simulink model "LSM_4p6U10_v01_06022022_NEW_ECC_2019a"  (R2019a)
settings: Solver=FixedStepAuto  StartTime=0.0  StopTime=Inf  FixedStep=Ts_lowspeed  RelTol=1e-3  EnableMultiTasking=on
PostLoadFcn:
  | , if any(exist('dsrtsu_mdlpostloadfcn', 'file') == [2, 3, 6]), try dsrtsu_mdlpostloadfcn('Execute', bdroot); catch fprintf('Error in PostLoadFcn (dsrtsu_mdlpostloadfcn) for model "%s":\n %s\n', bdroot, lasterr); end, end,
values from neighbouring files (symbols this model uses):
  Ts_lowspeed = 0.05    [Parameters_4p6U10.m]
undefined symbols (not defined in the file or in its folder): Down, GPTRIP1SEL, GPTRIP2SEL, TZ1, TZ2, Up
libraries: simulink x91, simulink_extras x25, c2802xlib x12, c2837xDlib x8, c280xlib x8
(part 2 of 2)

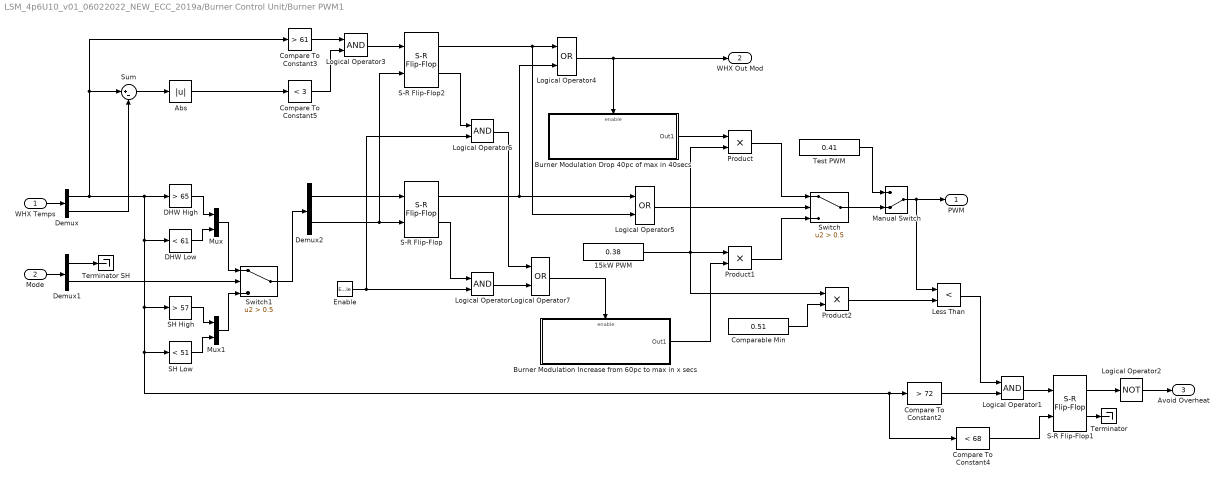
== system LSM_4p6U10_v01_06022022_NEW_ECC_2019a/Burner Control Unit/Burner PWM1 ==
  WHX Temps : Inport
  Mode : Inport  Port=2
  Enable : EnablePort  StatesWhenEnabling=reset  ShowOutputPort=on
  15kW PWM : Constant  Value=0.38  OutDataTypeStr=double
  Abs : Abs
  Burner Modulation Drop 40pc of max in 40secs : Subsystem
  Burner Modulation Increase from 60pc to max in x secs : Subsystem
  Comparable Min : Constant  Value=0.51  OutDataTypeStr=double
  Compare To Constant2 : simulink/Logic and Bit Operations/Compare To Constant  relop=>  const=72  OutDataTypeStr=boolean
  Compare To Constant3 : simulink/Logic and Bit Operations/Compare To Constant  relop=>  const=61  OutDataTypeStr=boolean
  Compare To Constant4 : simulink/Logic and Bit Operations/Compare To Constant  relop=<  const=68  OutDataTypeStr=boolean
  Compare To Constant5 : simulink/Logic and Bit Operations/Compare To Constant  relop=<  const=3  OutDataTypeStr=boolean
  DHW High : simulink/Logic and Bit Operations/Compare To Constant  relop=>  const=65  OutDataTypeStr=boolean
  DHW Low : simulink/Logic and Bit Operations/Compare To Constant  relop=<  const=61  OutDataTypeStr=boolean
  Demux : Demux  Outputs=2
  Demux1 : Demux  Outputs=2
  Demux2 : Demux  Outputs=2
  Less Than : RelationalOperator  Operator=<  OutDataTypeStr=boolean  RndMeth=Simplest
  Logical Operator{,1,3,6} (4 alike) : Logic  AllPortsSameDT=off  OutDataTypeStr=boolean
  Logical Operator2 : Logic  Operator=NOT  AllPortsSameDT=off  OutDataTypeStr=boolean
  Logical Operator4 : Logic  Operator=OR  AllPortsSameDT=off  OutDataTypeStr=boolean
  Logical Operator5 : Logic  Operator=OR  AllPortsSameDT=off  OutDataTypeStr=boolean
  Logical Operator7 : Logic  Operator=OR  AllPortsSameDT=off  OutDataTypeStr=boolean
  Manual Switch : ManualSwitch  CurrentSetting=0
  Mux : Mux  Inputs=2
  Mux1 : Mux  Inputs=2
  Product : Product
  Product1 : Product
  Product2 : Product
  S-R Flip-Flop : simulink_extras/Flip Flops/S-R Flip-Flop  initial_condition=0
  S-R Flip-Flop1 : simulink_extras/Flip Flops/S-R Flip-Flop  initial_condition=0
  S-R Flip-Flop2 : simulink_extras/Flip Flops/S-R Flip-Flop  initial_condition=0
  SH High : simulink/Logic and Bit Operations/Compare To Constant  relop=>  const=57  OutDataTypeStr=boolean
  SH Low : simulink/Logic and Bit Operations/Compare To Constant  relop=<  const=51  OutDataTypeStr=boolean
  Sum : Sum  Inputs=|+-
  Switch : Switch  Criteria=u2 > Threshold  Threshold=0.5
  Switch1 : Switch  Criteria=u2 > Threshold  Threshold=0.5
  Terminator : Terminator
  Terminator SH : Terminator
  Test PWM : Constant  Value=0.41  OutDataTypeStr=double
  PWM : Outport  VectorParamsAs1DForOutWhenUnconnected=on
  WHX Out Mod : Outport  Port=2  VectorParamsAs1DForOutWhenUnconnected=on
  Avoid Overheat : Outport  Port=3  VectorParamsAs1DForOutWhenUnconnected=on
  wires:
  Product2/1 -> Less Than/2
  Comparable Min/1 -> Product2/2
  Compare To Constant4/1 -> S-R Flip-Flop1/2
  Logical Operator2/1 -> Avoid Overheat/1
  S-R Flip-Flop1/1 -> Logical Operator2/1
  S-R Flip-Flop1/2 -> Terminator/1
  Logical Operator1/1 -> S-R Flip-Flop1/1
  Less Than/1 -> Logical Operator1/1
  Compare To Constant2/1 -> Logical Operator1/2
  Test PWM/1 -> Manual Switch/1
  Switch/1 -> Manual Switch/2
  Logical Operator/1 -> Logical Operator7/2
  Enable/1 -> Logical Operator6/2, Logical Operator/2
  Product1/1 -> Switch/3
  Burner Modulation Increase from 60pc to max in x secs/1(Out1) -> Product1/2
  Product/1 -> Switch/1
  Burner Modulation Drop 40pc of max in 40secs/1(Out1) -> Product/1
  Demux2/2 -> S-R Flip-Flop2/2, S-R Flip-Flop/2
  Manual Switch/1 -> PWM/1, Less Than/1
  S-R Flip-Flop/2 -> Logical Operator/1
  S-R Flip-Flop/1 -> Logical Operator5/1, Logical Operator4/2
  Demux2/1 -> S-R Flip-Flop/1
  Demux/1 -> DHW High/1, DHW Low/1, Compare To Constant2/1, Compare To Constant4/1, SH Low/1, SH High/1, Compare To Constant3/1, Sum/1
  15kW PWM/1 -> Product2/1, Product/2, Product1/1
  WHX Temps/1 -> Demux/1
  Demux/2 -> Sum/2
  Sum/1 -> Abs/1
  Abs/1 -> Compare To Constant5/1
  Compare To Constant3/1 -> Logical Operator3/1
  Compare To Constant5/1 -> Logical Operator3/2
  Logical Operator3/1 -> S-R Flip-Flop2/1
  S-R Flip-Flop2/1 -> Logical Operator5/2, Logical Operator4/1
  Logical Operator4/1 -> Burner Modulation Drop 40pc of max in 40secs/Enable, WHX Out Mod/1
  S-R Flip-Flop2/2 -> Logical Operator6/1
  Logical Operator5/1 -> Switch/2
  Logical Operator7/1 -> Burner Modulation Increase from 60pc to max in x secs/Enable
  Logical Operator6/1 -> Logical Operator7/1
  Mode/1 -> Demux1/1
  Demux1/1 -> Terminator SH/1
  Demux1/2 -> Switch1/2
  DHW High/1 -> Mux/1
  DHW Low/1 -> Mux/2
  SH High/1 -> Mux1/1
  SH Low/1 -> Mux1/2
  Mux1/1 -> Switch1/3
  Mux/1 -> Switch1/1
  Switch1/1 -> Demux2/1

== system LSM_4p6U10_v01_06022022_NEW_ECC_2019a/Burner Control Unit/Emergency Burner Shut Off ==
  Max HHT Temp : Inport
  Boolean 0 : Constant  Value=0  OutDataTypeStr=boolean
  Boolean 1 : Constant  OutDataTypeStr=boolean
  Boolean 14 : Constant  OutDataTypeStr=boolean
  Boolean 15 : Constant  Value=0  OutDataTypeStr=boolean
  Data Type Conversion : DataTypeConversion  OutDataTypeStr=double
  Emergency Shut Off T3 : Switch  Criteria=u2 > Threshold  Threshold=615
  Logical Operator : Logic  Operator=NOT  AllPortsSameDT=off  OutDataTypeStr=boolean
  S-R Flip-Flop : simulink_extras/Flip Flops/S-R Flip-Flop  initial_condition=0
  T3 Temp TH Reset : Switch  Criteria=u2 > Threshold  Threshold=450
  Terminator : Terminator
  Shut Off Command : Outport  VectorParamsAs1DForOutWhenUnconnected=on
  Emergency Shut OFF BL : Outport  Port=2  VectorParamsAs1DForOutWhenUnconnected=on
  wires:
  Boolean 1/1 -> Emergency Shut Off T3/1
  Boolean 0/1 -> Emergency Shut Off T3/3
  Emergency Shut Off T3/1 -> S-R Flip-Flop/1
  S-R Flip-Flop/1 -> Emergency Shut OFF BL/1, Logical Operator/1
  S-R Flip-Flop/2 -> Terminator/1
  T3 Temp TH Reset/1 -> S-R Flip-Flop/2
  Max HHT Temp/1 -> T3 Temp TH Reset/2, Emergency Shut Off T3/2
  Boolean 15/1 -> T3 Temp TH Reset/1
  Boolean 14/1 -> T3 Temp TH Reset/3
  Logical Operator/1 -> Data Type Conversion/1
  Data Type Conversion/1 -> Shut Off Command/1

== system LSM_4p6U10_v01_06022022_NEW_ECC_2019a/Burner Control Unit/Protected Modulation Drop 25pc of max in 50s ==
  Enable : EnablePort  StatesWhenEnabling=reset
  Constant : Constant
  Gain : Gain  Gain=-0.0025
  Integrator : Integrator  LimitOutput=on  UpperSaturationLimit=300  LowerSaturationLimit=0
  Limit Saturation : Saturate  UpperLimit=1  LowerLimit=0.75
  Sum : Sum  Inputs=|++
  Unit : Constant
  Out1 : Outport  VectorParamsAs1DForOutWhenUnconnected=on
  wires:
  Constant/1 -> Integrator/1
  Integrator/1 -> Gain/1
  Gain/1 -> Sum/1
  Unit/1 -> Sum/2
  Sum/1 -> Limit Saturation/1
  Limit Saturation/1 -> Out1/1

== system LSM_4p6U10_v01_06022022_NEW_ECC_2019a/Burner Control Unit/Reduction of Max PWM ==
  Max HHX Temp : Inport
  Boolean 0 : Constant  Value=0  OutDataTypeStr=boolean
  Boolean 1 : Constant  OutDataTypeStr=boolean
  Boolean 14 : Constant  OutDataTypeStr=boolean
  Boolean 15 : Constant  Value=0  OutDataTypeStr=boolean
  Emergency Shut Off T3 : Switch  Criteria=u2 > Threshold  Threshold=600
  S-R Flip-Flop : simulink_extras/Flip Flops/S-R Flip-Flop  initial_condition=0
  T3 Temp TH Reset : Switch  Criteria=u2 > Threshold  Threshold=580
  Terminator : Terminator
  Boolean 1 For Protection : Outport  VectorParamsAs1DForOutWhenUnconnected=on
  wires:
  Boolean 1/1 -> Emergency Shut Off T3/1
  Boolean 0/1 -> Emergency Shut Off T3/3
  Emergency Shut Off T3/1 -> S-R Flip-Flop/1
  S-R Flip-Flop/2 -> Terminator/1
  T3 Temp TH Reset/1 -> S-R Flip-Flop/2
  Max HHX Temp/1 -> T3 Temp TH Reset/2, Emergency Shut Off T3/2
  Boolean 15/1 -> T3 Temp TH Reset/1
  Boolean 14/1 -> T3 Temp TH Reset/3
  S-R Flip-Flop/1 -> Boolean 1 For Protection/1

== system LSM_4p6U10_v01_06022022_NEW_ECC_2019a/Flame Sense Relative to Motion/FLAME LOSS DECISION ==
  Enable : EnablePort  StatesWhenEnabling=reset
  0 to 91 : Integrator  LimitOutput=on  UpperSaturationLimit=91  LowerSaturationLimit=0
  Compare To Constant : simulink/Logic and Bit Operations/Compare To Constant  relop=>  const=90  OutDataTypeStr=boolean
  Constant : Constant
  Out1 : Outport
  wires:
  0 to 91/1 -> Compare To Constant/1
  Constant/1 -> 0 to 91/1
  Compare To Constant/1 -> Out1/1

== system LSM_4p6U10_v01_06022022_NEW_ECC_2019a/Pump Commands FIELD INSTALLATION/Conversion for micro ==
  WHXPC : Inport
  CHXPC : Inport  Port=2
  Ceil2 : Rounding  Operator=ceil
  Ceil4 : Rounding  Operator=ceil
  "Convert Volts to 0-1 Command " : Gain  Gain=1/10
  Convert Volts to 0-1 Command : Gain  Gain=1/10
  Convert to uint1 : DataTypeConversion  OutDataTypeStr=uint16
  Convert to uint16 : DataTypeConversion  OutDataTypeStr=uint16
  Gain2 : Gain  Gain=1023
  Gain3 : Gain  Gain=1023
  CHX Pump : Outport
  WHX Pump : Outport  Port=2
  wires:
  Ceil4/1 -> Convert to uint1/1
  Ceil2/1 -> Convert to uint16/1
  Convert to uint16/1 -> CHX Pump/1  "CHX Pump"
  Gain3/1 -> Ceil2/1
  Convert to uint1/1 -> WHX Pump/1  "WHX Pump"
  "Convert Volts to 0-1 Command "/1 -> Gain2/1
  Convert Volts to 0-1 Command/1 -> Gain3/1
  CHXPC/1 -> "Convert Volts to 0-1 Command "/1
  Gain2/1 -> Ceil4/1
  WHXPC/1 -> Convert Volts to 0-1 Command/1

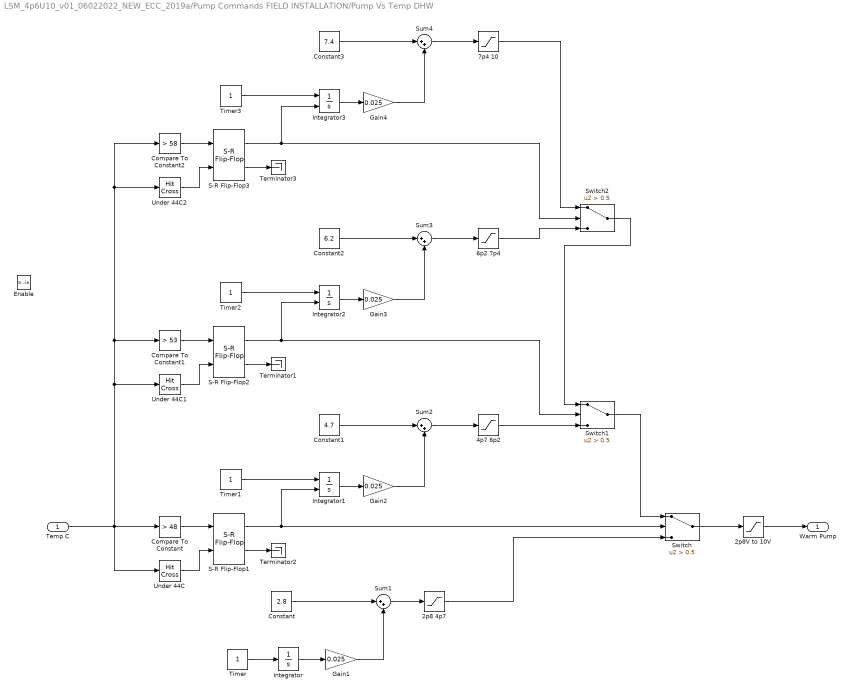
== system LSM_4p6U10_v01_06022022_NEW_ECC_2019a/Pump Commands FIELD INSTALLATION/Pump Vs Temp DHW ==
  Temp C : Inport
  Enable : EnablePort  StatesWhenEnabling=reset
  2p8 4p7 : Saturate  UpperLimit=4.7  LowerLimit=2.8
  2p8V to 10V : Saturate  UpperLimit=10  LowerLimit=2.8
  4p7 6p2 : Saturate  UpperLimit=6.2  LowerLimit=4.7
  6p2 7p4 : Saturate  UpperLimit=7.4  LowerLimit=6.2
  7p4 10 : Saturate  UpperLimit=10  LowerLimit=7.4
  Compare To Constant : simulink/Logic and Bit Operations/Compare To Constant  relop=>  const=48  OutDataTypeStr=boolean
  Compare To Constant1 : simulink/Logic and Bit Operations/Compare To Constant  relop=>  const=53  OutDataTypeStr=boolean
  Compare To Constant2 : simulink/Logic and Bit Operations/Compare To Constant  relop=>  const=58  OutDataTypeStr=boolean
  Constant : Constant  Value=2.8
  Constant1 : Constant  Value=4.7
  Constant2 : Constant  Value=6.2
  Constant3 : Constant  Value=7.4
  Gain{1..4} (4 alike) : Gain  Gain=0.025
  Integrator : Integrator  LimitOutput=on  UpperSaturationLimit=300  LowerSaturationLimit=0
  Integrator1 : Integrator  ExternalReset=rising  LimitOutput=on  UpperSaturationLimit=300  LowerSaturationLimit=0
  Integrator2 : Integrator  ExternalReset=rising  LimitOutput=on  UpperSaturationLimit=300  LowerSaturationLimit=0
  Integrator3 : Integrator  ExternalReset=rising  LimitOutput=on  UpperSaturationLimit=300  LowerSaturationLimit=0
  S-R Flip-Flop1 : simulink_extras/Flip Flops/S-R Flip-Flop  initial_condition=0
  S-R Flip-Flop2 : simulink_extras/Flip Flops/S-R Flip-Flop  initial_condition=0
  S-R Flip-Flop3 : simulink_extras/Flip Flops/S-R Flip-Flop  initial_condition=0
  Sum{1..4} (4 alike) : Sum  Inputs=|++
  Switch : Switch  Criteria=u2 > Threshold  Threshold=0.5
  Switch1 : Switch  Criteria=u2 > Threshold  Threshold=0.5
  Switch2 : Switch  Criteria=u2 > Threshold  Threshold=0.5
  Terminator1 : Terminator
  Terminator2 : Terminator
  Terminator3 : Terminator
  Timer{,1..3} (4 alike) : Constant
  Under 44C : HitCross  HitCrossingOffset=40  HitCrossingDirection=falling
  Under 44C1 : HitCross  HitCrossingOffset=40  HitCrossingDirection=falling
  Under 44C2 : HitCross  HitCrossingOffset=40  HitCrossingDirection=falling
  Warm Pump : Outport  VectorParamsAs1DForOutWhenUnconnected=on
  wires:
  2p8V to 10V/1 -> Warm Pump/1
  S-R Flip-Flop1/2 -> Terminator2/1
  Under 44C/1 -> S-R Flip-Flop1/2
  Compare To Constant/1 -> S-R Flip-Flop1/1
  S-R Flip-Flop1/1 -> Switch/2, Integrator1/2
  Constant/1 -> Sum1/1
  Gain1/1 -> Sum1/2
  Sum1/1 -> 2p8 4p7/1
  Integrator/1 -> Gain1/1
  Timer/1 -> Integrator/1
  2p8 4p7/1 -> Switch/3
  Gain2/1 -> Sum2/2
  Integrator1/1 -> Gain2/1
  Constant1/1 -> Sum2/1
  Timer1/1 -> Integrator1/1
  4p7 6p2/1 -> Switch1/3
  Sum2/1 -> 4p7 6p2/1
  Switch1/1 -> Switch/1
  Switch/1 -> 2p8V to 10V/1
  6p2 7p4/1 -> Switch2/3
  Sum3/1 -> 6p2 7p4/1
  Timer2/1 -> Integrator2/1
  Integrator2/1 -> Gain3/1
  S-R Flip-Flop2/1 -> Switch1/2, Integrator2/2
  S-R Flip-Flop2/2 -> Terminator1/1
  Compare To Constant1/1 -> S-R Flip-Flop2/1
  Constant2/1 -> Sum3/1
  Under 44C1/1 -> S-R Flip-Flop2/2
  Gain3/1 -> Sum3/2
  S-R Flip-Flop3/2 -> Terminator3/1
  Under 44C2/1 -> S-R Flip-Flop3/2
  S-R Flip-Flop3/1 -> Switch2/2, Integrator3/2
  Compare To Constant2/1 -> S-R Flip-Flop3/1
  Constant3/1 -> Sum4/1
  Sum4/1 -> 7p4 10/1
  Integrator3/1 -> Gain4/1
  7p4 10/1 -> Switch2/1
  Temp C/1 -> Compare To Constant2/1, Under 44C2/1, Compare To Constant1/1, Under 44C1/1, Under 44C/1, Compare To Constant/1
  Gain4/1 -> Sum4/2
  Timer3/1 -> Integrator3/1
  Switch2/1 -> Switch1/1

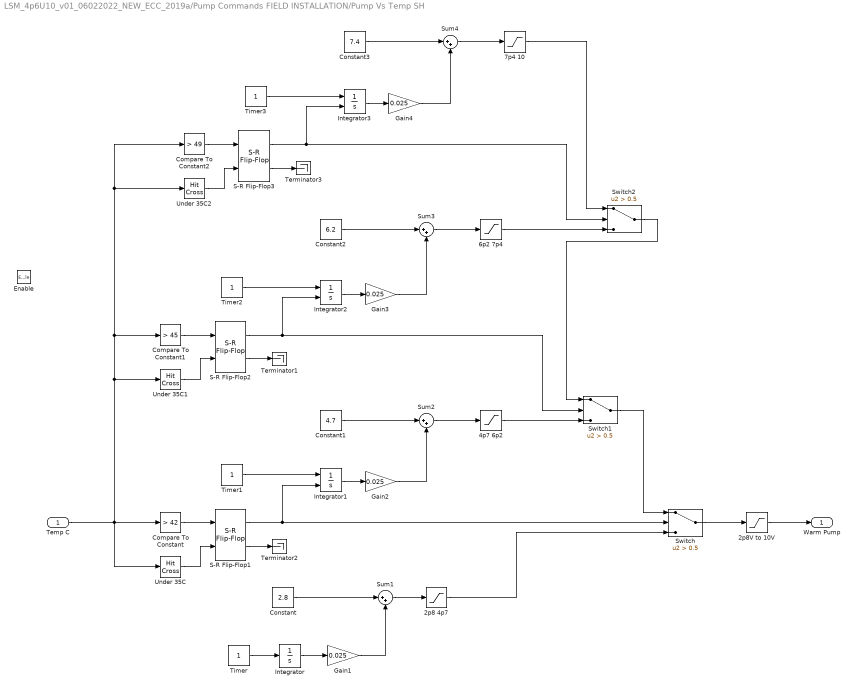
== system LSM_4p6U10_v01_06022022_NEW_ECC_2019a/Pump Commands FIELD INSTALLATION/Pump Vs Temp SH ==
  Temp C : Inport
  Enable : EnablePort  StatesWhenEnabling=reset
  2p8 4p7 : Saturate  UpperLimit=4.7  LowerLimit=2.8
  2p8V to 10V : Saturate  UpperLimit=10  LowerLimit=2.8
  4p7 6p2 : Saturate  UpperLimit=6.2  LowerLimit=4.7
  6p2 7p4 : Saturate  UpperLimit=7.4  LowerLimit=6.2
  7p4 10 : Saturate  UpperLimit=10  LowerLimit=7.4
  Compare To Constant : simulink/Logic and Bit Operations/Compare To Constant  relop=>  const=42  OutDataTypeStr=boolean
  Compare To Constant1 : simulink/Logic and Bit Operations/Compare To Constant  relop=>  const=45  OutDataTypeStr=boolean
  Compare To Constant2 : simulink/Logic and Bit Operations/Compare To Constant  relop=>  const=49  OutDataTypeStr=boolean
  Constant : Constant  Value=2.8
  Constant1 : Constant  Value=4.7
  Constant2 : Constant  Value=6.2
  Constant3 : Constant  Value=7.4
  Gain{1..4} (4 alike) : Gain  Gain=0.025
  Integrator : Integrator  LimitOutput=on  UpperSaturationLimit=300  LowerSaturationLimit=0
  Integrator1 : Integrator  ExternalReset=rising  LimitOutput=on  UpperSaturationLimit=300  LowerSaturationLimit=0
  Integrator2 : Integrator  ExternalReset=rising  LimitOutput=on  UpperSaturationLimit=300  LowerSaturationLimit=0
  Integrator3 : Integrator  ExternalReset=rising  LimitOutput=on  UpperSaturationLimit=300  LowerSaturationLimit=0
  S-R Flip-Flop1 : simulink_extras/Flip Flops/S-R Flip-Flop  initial_condition=0
  S-R Flip-Flop2 : simulink_extras/Flip Flops/S-R Flip-Flop  initial_condition=0
  S-R Flip-Flop3 : simulink_extras/Flip Flops/S-R Flip-Flop  initial_condition=0
  Sum{1..4} (4 alike) : Sum  Inputs=|++
  Switch : Switch  Criteria=u2 > Threshold  Threshold=0.5
  Switch1 : Switch  Criteria=u2 > Threshold  Threshold=0.5
  Switch2 : Switch  Criteria=u2 > Threshold  Threshold=0.5
  Terminator1 : Terminator
  Terminator2 : Terminator
  Terminator3 : Terminator
  Timer{,1..3} (4 alike) : Constant
  Under 35C : HitCross  HitCrossingOffset=35  HitCrossingDirection=falling
  Under 35C1 : HitCross  HitCrossingOffset=35  HitCrossingDirection=falling
  Under 35C2 : HitCross  HitCrossingOffset=35  HitCrossingDirection=falling
  Warm Pump : Outport  VectorParamsAs1DForOutWhenUnconnected=on
  wires:
  2p8V to 10V/1 -> Warm Pump/1
  S-R Flip-Flop1/2 -> Terminator2/1
  Under 35C/1 -> S-R Flip-Flop1/2
  Compare To Constant/1 -> S-R Flip-Flop1/1
  S-R Flip-Flop1/1 -> Switch/2, Integrator1/2
  Constant/1 -> Sum1/1
  Gain1/1 -> Sum1/2
  Sum1/1 -> 2p8 4p7/1
  Integrator/1 -> Gain1/1
  Timer/1 -> Integrator/1
  2p8 4p7/1 -> Switch/3
  Gain2/1 -> Sum2/2
  Integrator1/1 -> Gain2/1
  Constant1/1 -> Sum2/1
  Timer1/1 -> Integrator1/1
  4p7 6p2/1 -> Switch1/3
  Sum2/1 -> 4p7 6p2/1
  Switch1/1 -> Switch/1
  Switch/1 -> 2p8V to 10V/1
  6p2 7p4/1 -> Switch2/3
  Sum3/1 -> 6p2 7p4/1
  Timer2/1 -> Integrator2/1
  Integrator2/1 -> Gain3/1
  S-R Flip-Flop2/1 -> Switch1/2, Integrator2/2
  S-R Flip-Flop2/2 -> Terminator1/1
  Compare To Constant1/1 -> S-R Flip-Flop2/1
  Constant2/1 -> Sum3/1
  Under 35C1/1 -> S-R Flip-Flop2/2
  Gain3/1 -> Sum3/2
  Constant3/1 -> Sum4/1
  Gain4/1 -> Sum4/2
  7p4 10/1 -> Switch2/1
  Under 35C2/1 -> S-R Flip-Flop3/2
  Integrator3/1 -> Gain4/1
  S-R Flip-Flop3/1 -> Switch2/2, Integrator3/2
  Temp C/1 -> Compare To Constant2/1, Under 35C2/1, Compare To Constant1/1, Under 35C1/1, Under 35C/1, Compare To Constant/1
  Compare To Constant2/1 -> S-R Flip-Flop3/1
  S-R Flip-Flop3/2 -> Terminator3/1
  Sum4/1 -> 7p4 10/1
  Timer3/1 -> Integrator3/1
  Switch2/1 -> Switch1/1

== system LSM_4p6U10_v01_06022022_NEW_ECC_2019a/Pump Commands FIELD INSTALLATION/Timer // Integrator 0-101s1 ==
  WPC : Inport
  Enable : EnablePort  StatesWhenEnabling=reset  ShowOutputPort=on
  Gain : Gain  Gain=-0.1
  Integrator : Integrator  ExternalReset=rising  LimitOutput=on  UpperSaturationLimit=300  LowerSaturationLimit=0
  Saturation : Saturate  UpperLimit=10  LowerLimit=2.8
  Sum : Sum  Inputs=|++
  Timer : Constant
  Out1 : Outport  VectorParamsAs1DForOutWhenUnconnected=on
  wires:
  Timer/1 -> Integrator/1
  Integrator/1 -> Gain/1
  Enable/1 -> Integrator/2
  Sum/1 -> Saturation/1
  WPC/1 -> Sum/1
  Gain/1 -> Sum/2
  Saturation/1 -> Out1/1

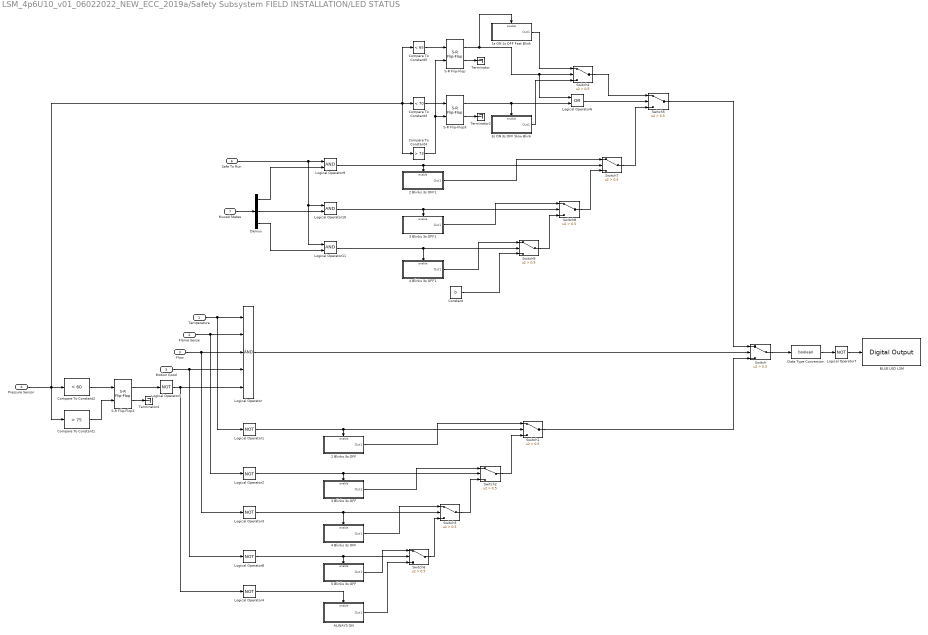
== system LSM_4p6U10_v01_06022022_NEW_ECC_2019a/Safety Subsystem FIELD INSTALLATION/LED STATUS ==
  Temperature : Inport
  Flame Sense : Inport  Port=2
  Flow : Inport  Port=3
  Pressure Sensor : Inport  Port=4
  Motion Good : Inport  Port=5
  Safe To Run : Inport  Port=6
  Muxed States : Inport  Port=7
  1s ON 1s OFF Fast Blink : Subsystem
  2 Blinks 3s OFF : Subsystem
  2 Blinks 3s OFF1 : Subsystem
  3 Blinks 3s OFF : Subsystem
  3 Blinks 3s OFF1 : Subsystem
  3s ON 3s OFF Slow Blink : Subsystem
  4 Blinks 3s OFF : Subsystem
  4 Blinks 3s OFF1 : Subsystem
  5 Blinks 3s OFF : Subsystem
  ALWAYS ON : Subsystem
  BLUE LED LSM : c2837xDlib/Digital Output  GPIO_Number=GPIO24~GPIO31  GPIO_Bit0=off  GPIO_BIT0_Toggle=off  GPIO_Bit1=off  GPIO_BIT1_Toggle=off  GPIO_Bit2=off  GPIO_BIT2_Toggle=off  GPIO_Bit3=off  GPIO_BIT3_Toggle=off  GPIO_Bit4=off  GPIO_BIT4_Toggle=off  GPIO_Bit5=off  GPIO_BIT5_Toggle=off  GPIO_Bit6=off  GPIO_BIT6_Toggle=off  GPIO_Bit7=on  GPIO_BIT7_Toggle=off
      settings: SourceProductBaseCode=TIC2000
  Compare To Constant1 : simulink/Logic and Bit Operations/Compare To Constant  relop=>  const=75  OutDataTypeStr=boolean
  Compare To Constant2 : simulink/Logic and Bit Operations/Compare To Constant  relop=<  const=60  OutDataTypeStr=boolean
  Compare To Constant3 : simulink/Logic and Bit Operations/Compare To Constant  relop=<  const=70  OutDataTypeStr=boolean
  Compare To Constant4 : simulink/Logic and Bit Operations/Compare To Constant  relop=>  const=73  OutDataTypeStr=boolean
  Compare To Constant5 : simulink/Logic and Bit Operations/Compare To Constant  relop=<  const=65  OutDataTypeStr=boolean
  Constant : Constant  Value=0  OutDataTypeStr=boolean
  Data Type Conversion : DataTypeConversion  OutDataTypeStr=boolean
  Demux : Demux  Outputs=3
  Logical Operator : Logic  Inputs=5  AllPortsSameDT=off  OutDataTypeStr=boolean
  Logical Operator{1..5,7..8} (7 alike) : Logic  Operator=NOT  AllPortsSameDT=off  OutDataTypeStr=boolean
  Logical Operator10 : Logic  AllPortsSameDT=off  OutDataTypeStr=boolean
  Logical Operator11 : Logic  AllPortsSameDT=off  OutDataTypeStr=boolean
  Logical Operator6 : Logic  Operator=OR  AllPortsSameDT=off  OutDataTypeStr=boolean
  Logical Operator9 : Logic  AllPortsSameDT=off  OutDataTypeStr=boolean
  S-R Flip-Flop : simulink_extras/Flip Flops/S-R Flip-Flop  initial_condition=0
  S-R Flip-Flop1 : simulink_extras/Flip Flops/S-R Flip-Flop  initial_condition=0
  S-R Flip-Flop3 : simulink_extras/Flip Flops/S-R Flip-Flop  initial_condition=0
  Switch{,1..9} (10 alike) : Switch  Criteria=u2 > Threshold  Threshold=0.5
  Terminator : Terminator
  Terminator2 : Terminator
  Terminator4 : Terminator
  wires:
  Temperature/1 -> Logical Operator1/1, Logical Operator/1
  Flame Sense/1 -> Logical Operator2/1, Logical Operator/2
  Flow/1 -> Logical Operator3/1, Logical Operator/3
  Logical Operator5/1 -> Logical Operator/5, Logical Operator4/1
  Logical Operator/1 -> Switch/2
  Logical Operator1/1 -> Switch1/2, 2 Blinks 3s OFF/Enable
  Logical Operator2/1 -> Switch2/2, 3 Blinks 3s OFF/Enable
  Logical Operator3/1 -> Switch3/2, 4 Blinks 3s OFF/Enable
  Logical Operator4/1 -> ALWAYS ON/Enable
  Compare To Constant1/1 -> S-R Flip-Flop1/2
  Compare To Constant2/1 -> S-R Flip-Flop1/1
  S-R Flip-Flop1/2 -> Terminator4/1
  S-R Flip-Flop1/1 -> Logical Operator5/1
  ALWAYS ON/1(Out1) -> Switch6/3
  Switch1/1 -> Switch/3
  2 Blinks 3s OFF/1(Out1) -> Switch1/1
  Switch2/1 -> Switch1/3
  3 Blinks 3s OFF/1(Out1) -> Switch2/1
  4 Blinks 3s OFF/1(Out1) -> Switch3/1
  Switch3/1 -> Switch2/3
  Compare To Constant5/1 -> S-R Flip-Flop/1
  3s ON 3s OFF Slow Blink/1(Out1) -> Switch4/3
  Compare To Constant4/1 -> S-R Flip-Flop/2, S-R Flip-Flop3/2
  Pressure Sensor/1 -> Compare To Constant4/1, Compare To Constant3/1, Compare To Constant5/1, Compare To Constant1/1, Compare To Constant2/1
  S-R Flip-Flop3/2 -> Terminator2/1
  Data Type Conversion/1 -> Logical Operator7/1
  1s ON 1s OFF Fast Blink/1(Out1) -> Switch4/1
  S-R Flip-Flop/1 -> 1s ON 1s OFF Fast Blink/Enable, Logical Operator6/1, Switch4/2
  S-R Flip-Flop/2 -> Terminator/1
  Compare To Constant3/1 -> S-R Flip-Flop3/1
  S-R Flip-Flop3/1 -> 3s ON 3s OFF Slow Blink/Enable, Logical Operator6/2
  Switch/1 -> Data Type Conversion/1
  Switch4/1 -> Switch5/1
  Switch5/1 -> Switch/1
  Logical Operator6/1 -> Switch5/2
  Logical Operator7/1 -> BLUE LED LSM/1
  Motion Good/1 -> Logical Operator8/1, Logical Operator/4
  Logical Operator8/1 -> 5 Blinks 3s OFF/Enable, Switch6/2
  5 Blinks 3s OFF/1(Out1) -> Switch6/1
  Switch6/1 -> Switch3/3
  Safe To Run/1 -> Logical Operator11/1, Logical Operator10/1, Logical Operator9/1
  Muxed States/1 -> Demux/1
  Demux/1 -> Logical Operator9/2
  Demux/2 -> Logical Operator10/2
  Demux/3 -> Logical Operator11/2
  Constant/1 -> Switch9/3
  2 Blinks 3s OFF1/1(Out1) -> Switch7/1
  Switch8/1 -> Switch7/3
  Switch9/1 -> Switch8/3
  4 Blinks 3s OFF1/1(Out1) -> Switch9/1
  Logical Operator9/1 -> Switch7/2, 2 Blinks 3s OFF1/Enable
  3 Blinks 3s OFF1/1(Out1) -> Switch8/1
  Logical Operator11/1 -> Switch9/2, 4 Blinks 3s OFF1/Enable
  Logical Operator10/1 -> Switch8/2, 3 Blinks 3s OFF1/Enable
  Switch7/1 -> Switch5/3

== system LSM_4p6U10_v01_06022022_NEW_ECC_2019a/Safety Subsystem FIELD INSTALLATION/Over 9s 1BL ==
  Enable : EnablePort  StatesWhenEnabling=reset
  Compare To Constant : simulink/Logic and Bit Operations/Compare To Constant  relop=>  const=9  OutDataTypeStr=boolean
  Constant : Constant
  Integrator : Integrator  LimitOutput=on  UpperSaturationLimit=11  LowerSaturationLimit=0
  Out1 : Outport
  wires:
  Constant/1 -> Integrator/1
  Integrator/1 -> Compare To Constant/1
  Compare To Constant/1 -> Out1/1

== system LSM_4p6U10_v01_06022022_NEW_ECC_2019a/TC Decision Making/TC Set 1 ==
  In1 : Inport
  In2 : Inport  Port=2
  Abs : Abs
  Compare To Constant : simulink/Logic and Bit Operations/Compare To Constant  relop=<  const=200  OutDataTypeStr=boolean
  Compare To Constant1 : simulink/Logic and Bit Operations/Compare To Constant  relop=>  const=850  OutDataTypeStr=boolean
  Compare To Constant2 : simulink/Logic and Bit Operations/Compare To Constant  relop=>  const=850  OutDataTypeStr=boolean
  Error Reading : Constant  Value=-10
  Logical Operator : Logic  AllPortsSameDT=off  OutDataTypeStr=boolean
  Priority Set 1 Offset to HiLimit : Constant  Value=40
  Relational Operator : RelationalOperator  OutDataTypeStr=boolean  RndMeth=Simplest
  Sum : Sum  Inputs=+-
  Sum2 : Sum  Inputs=|++
  Switch : Switch  Criteria=u2 > Threshold  Threshold=0.5
  Switch1 : Switch  Criteria=u2 > Threshold  Threshold=0.5
  Switch2 : Switch  Criteria=u2 > Threshold  Threshold=0.5
  High or neg10C Set 1 : Outport
  wires:
  In1/1 -> Compare To Constant1/1, Switch/1, Relational Operator/1, Sum/1
  In2/1 -> Compare To Constant2/1, Switch/3, Relational Operator/2, Sum/2
  Sum/1 -> Abs/1
  Abs/1 -> Compare To Constant/1
  Compare To Constant/1 -> Switch1/2
  Relational Operator/1 -> Switch/2
  Switch1/1 -> Switch2/3
  Error Reading/1 -> Switch2/1, Switch1/3
  Switch/1 -> Sum2/1
  Sum2/1 -> Switch1/1
  Priority Set 1 Offset to HiLimit/1 -> Sum2/2
  Compare To Constant2/1 -> Logical Operator/2
  Compare To Constant1/1 -> Logical Operator/1
  Logical Operator/1 -> Switch2/2
  Switch2/1 -> High or neg10C Set 1/1

== system LSM_4p6U10_v01_06022022_NEW_ECC_2019a/TC Decision Making/TC Set 2 ==
  In1 : Inport
  In2 : Inport  Port=2
  Abs : Abs
  Compare To Constant : simulink/Logic and Bit Operations/Compare To Constant  relop=<  const=200  OutDataTypeStr=boolean
  Compare To Constant1 : simulink/Logic and Bit Operations/Compare To Constant  relop=>  const=850  OutDataTypeStr=boolean
  Compare To Constant2 : simulink/Logic and Bit Operations/Compare To Constant  relop=>  const=850  OutDataTypeStr=boolean
  Error Reading : Constant  Value=-10
  Logical Operator : Logic  AllPortsSameDT=off  OutDataTypeStr=boolean
  Priority Set 2 Offset to HiLimit : Constant  Value=10
  Relational Operator : RelationalOperator  OutDataTypeStr=boolean  RndMeth=Simplest
  Sum : Sum  Inputs=+-
  Sum2 : Sum  Inputs=|++
  Switch : Switch  Criteria=u2 > Threshold  Threshold=0.5
  Switch1 : Switch  Criteria=u2 > Threshold  Threshold=0.5
  Switch2 : Switch  Criteria=u2 > Threshold  Threshold=0.5
  High or neg10C Set 2 : Outport
  wires:
  Compare To Constant/1 -> Switch1/2
  Relational Operator/1 -> Switch/2
  Sum/1 -> Abs/1
  Abs/1 -> Compare To Constant/1
  Sum2/1 -> Switch1/1
  Switch/1 -> Sum2/1
  Priority Set 2 Offset to HiLimit/1 -> Sum2/2
  Switch2/1 -> High or neg10C Set 2/1
  Switch1/1 -> Switch2/3
  Compare To Constant2/1 -> Logical Operator/2
  Error Reading/1 -> Switch2/1, Switch1/3
  Compare To Constant1/1 -> Logical Operator/1
  Logical Operator/1 -> Switch2/2
  In1/1 -> Compare To Constant1/1, Switch/1, Relational Operator/1, Sum/1
  In2/1 -> Compare To Constant2/1, Switch/3, Relational Operator/2, Sum/2

== system LSM_4p6U10_v01_06022022_NEW_ECC_2019a/TC Decision Making/TC Set 3 ==
  In1 : Inport
  In2 : Inport  Port=2
  Abs : Abs
  Compare To Constant : simulink/Logic and Bit Operations/Compare To Constant  relop=<  const=200  OutDataTypeStr=boolean
  Compare To Constant1 : simulink/Logic and Bit Operations/Compare To Constant  relop=>  const=850  OutDataTypeStr=boolean
  Compare To Constant2 : simulink/Logic and Bit Operations/Compare To Constant  relop=>  const=850  OutDataTypeStr=boolean
  Error Reading : Constant  Value=-10
  Logical Operator : Logic  AllPortsSameDT=off  OutDataTypeStr=boolean
  Priority Set 3 Offset to HiLimit : Constant  Value=-10
  Relational Operator : RelationalOperator  OutDataTypeStr=boolean  RndMeth=Simplest
  Sum : Sum  Inputs=+-
  Sum2 : Sum  Inputs=|++
  Switch : Switch  Criteria=u2 > Threshold  Threshold=0.5
  Switch1 : Switch  Criteria=u2 > Threshold  Threshold=0.5
  Switch2 : Switch  Criteria=u2 > Threshold  Threshold=0.5
  High or neg10C Set 3 : Outport
  wires:
  Compare To Constant/1 -> Switch1/2
  Relational Operator/1 -> Switch/2
  Sum/1 -> Abs/1
  Abs/1 -> Compare To Constant/1
  Sum2/1 -> Switch1/1
  Switch/1 -> Sum2/1
  Priority Set 3 Offset to HiLimit/1 -> Sum2/2
  Switch2/1 -> High or neg10C Set 3/1
  Switch1/1 -> Switch2/3
  Compare To Constant2/1 -> Logical Operator/2
  Error Reading/1 -> Switch2/1, Switch1/3
  Compare To Constant1/1 -> Logical Operator/1
  Logical Operator/1 -> Switch2/2
  In1/1 -> Compare To Constant1/1, Switch/1, Relational Operator/1, Sum/1
  In2/1 -> Compare To Constant2/1, Switch/3, Relational Operator/2, Sum/2

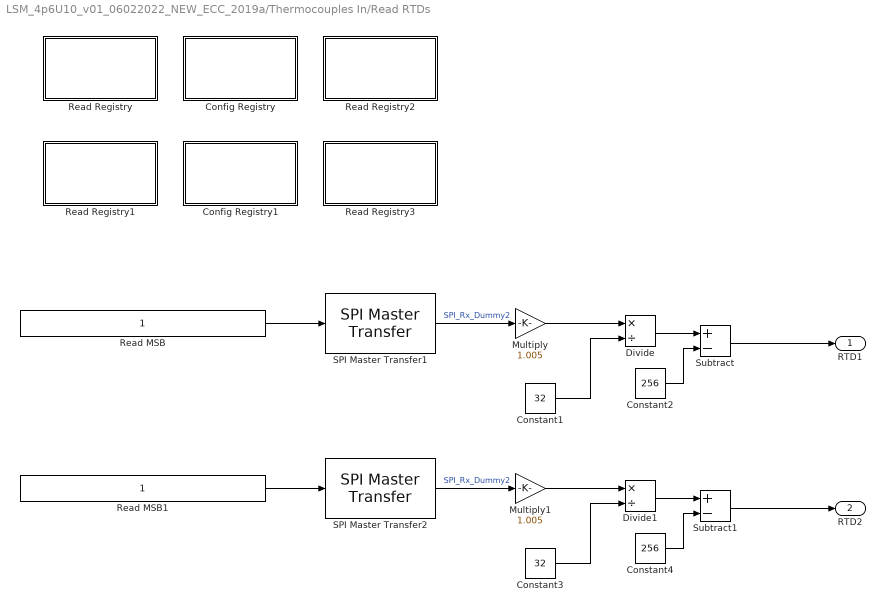
== system LSM_4p6U10_v01_06022022_NEW_ECC_2019a/Thermocouples In/Read RTDs ==
  Config Registry : Subsystem
  Config Registry1 : Subsystem
  Constant1 : Constant  Value=32
  Constant2 : Constant  Value=256
  Constant3 : Constant  Value=32
  Constant4 : Constant  Value=256
  Divide : Product  Inputs=*/
  Divide1 : Product  Inputs=*/
  Multiply : Gain  Gain=1.005
  Multiply1 : Gain  Gain=1.005
  Read MSB : Constant  OutDataTypeStr=uint16  SampleTime=-1
  Read MSB1 : Constant  OutDataTypeStr=uint16  SampleTime=-1
  Read Registry : Subsystem
  Read Registry1 : Subsystem
  Read Registry2 : Subsystem
  Read Registry3 : Subsystem
  SPI Master Transfer1 : c280xlib/SPI Master Transfer  SPISelect=SPI_A  ClockPolarity=Falling_edge  ClockPhase=Delay_half_cycle  SPIModule=uint32(0)  Mode=Master  BusSpeed=uint32(1000000)  FirstBitToTransfer=Most significant bit (MSB)  ClockMode=0  BlockFunction=Transfer  EnableRegisterAddress=on  RegisterAddress=1  OutputDataType=int8  OutputDataLength=1  DataBits=16  UseCustomSSPin=Explicit GPIO calls  ActiveLowSSPin=Active low  Pin=125
      settings: SourceProductName=Embedded Coder Support Package for Texas Instruments C2000 Processors
  SPI Master Transfer2 : c280xlib/SPI Master Transfer  SPISelect=SPI_A  ClockPolarity=Falling_edge  ClockPhase=Delay_half_cycle  SPIModule=uint32(0)  Mode=Master  BusSpeed=uint32(1000000)  FirstBitToTransfer=Most significant bit (MSB)  ClockMode=0  BlockFunction=Transfer  EnableRegisterAddress=on  RegisterAddress=1  OutputDataType=int8  OutputDataLength=1  DataBits=16  UseCustomSSPin=Explicit GPIO calls  ActiveLowSSPin=Active low  Pin=124
      settings: SourceProductName=Embedded Coder Support Package for Texas Instruments C2000 Processors
  Subtract : Sum  Inputs=+-
  Subtract1 : Sum  Inputs=+-
  RTD1 : Outport
  RTD2 : Outport  Port=2
  wires:
  Constant1/1 -> Divide/2
  Divide/1 -> Subtract/1
  Constant2/1 -> Subtract/2
  Subtract/1 -> RTD1/1
  Multiply/1 -> Divide/1
  Subtract1/1 -> RTD2/1
  Divide1/1 -> Subtract1/1
  Multiply1/1 -> Divide1/1
  Constant4/1 -> Subtract1/2
  Constant3/1 -> Divide1/2
  SPI Master Transfer1/1 -> Multiply/1  "SPI_Rx_Dummy2"
  Read MSB/1 -> SPI Master Transfer1/1
  SPI Master Transfer2/1 -> Multiply1/1  "SPI_Rx_Dummy2"
  Read MSB1/1 -> SPI Master Transfer2/1

== system LSM_4p6U10_v01_06022022_NEW_ECC_2019a/Burner Control Unit/Burner PWM1/Burner Modulation Drop 40pc of max in 40secs ==
  Enable : EnablePort  StatesWhenEnabling=reset
  Constant : Constant
  Gain : Gain  Gain=-0.0025
  Integrator : Integrator  LimitOutput=on  UpperSaturationLimit=500  LowerSaturationLimit=0
  Limit Saturation : Saturate  UpperLimit=1  LowerLimit=0.5
  Sum : Sum  Inputs=|++
  Unit : Constant
  Out1 : Outport  VectorParamsAs1DForOutWhenUnconnected=on
  wires:
  Limit Saturation/1 -> Out1/1
  Sum/1 -> Limit Saturation/1
  Unit/1 -> Sum/2
  Gain/1 -> Sum/1
  Integrator/1 -> Gain/1
  Constant/1 -> Integrator/1

== system LSM_4p6U10_v01_06022022_NEW_ECC_2019a/Burner Control Unit/Burner PWM1/Burner Modulation Increase from 60pc to max in x secs ==
  Enable : EnablePort  StatesWhenEnabling=reset
  Constant : Constant
  Gain : Gain  Gain=0.0025
  Integrator : Integrator  LimitOutput=on  UpperSaturationLimit=500  LowerSaturationLimit=0
  Limit Saturation : Saturate  UpperLimit=1  LowerLimit=0.5
  Sum : Sum  Inputs=|++
  Unit : Constant  Value=0.5
  Out1 : Outport  VectorParamsAs1DForOutWhenUnconnected=on
  wires:
  Constant/1 -> Integrator/1
  Integrator/1 -> Gain/1
  Gain/1 -> Sum/1
  Unit/1 -> Sum/2
  Sum/1 -> Limit Saturation/1
  Limit Saturation/1 -> Out1/1

== system LSM_4p6U10_v01_06022022_NEW_ECC_2019a/Safety Subsystem FIELD INSTALLATION/LED STATUS/1s ON 1s OFF Fast Blink ==
  Enable : EnablePort  StatesWhenEnabling=reset
  Pulse Generator : DiscretePulseGenerator  PulseType=Time based  PulseWidth=50
  Saturation : Saturate  UpperLimit=1  LowerLimit=0
  Out1 : Outport
  wires:
  Saturation/1 -> Out1/1
  Pulse Generator/1 -> Saturation/1

== system LSM_4p6U10_v01_06022022_NEW_ECC_2019a/Safety Subsystem FIELD INSTALLATION/LED STATUS/2 Blinks 3s OFF ==
  Enable : EnablePort  StatesWhenEnabling=reset
  Compare To Constant : simulink/Logic and Bit Operations/Compare To Constant  relop=<  const=0.25  OutDataTypeStr=boolean
  Compare To Constant1 : simulink/Logic and Bit Operations/Compare To Constant  relop=>  const=3.5  OutDataTypeStr=boolean
  Compare To Constant2 : simulink/Logic and Bit Operations/Compare To Constant  relop=<  const=0.85  OutDataTypeStr=boolean
  Constant : Constant
  Delay : Delay  DelayLength=1
  Integrator : Integrator  ExternalReset=rising  LimitOutput=on  UpperSaturationLimit=3.6  LowerSaturationLimit=0
  Switch : Switch  Criteria=u2 > Threshold  Threshold=0.5
  Out1 : Outport
  wires:
  Constant/1 -> Integrator/1
  Integrator/1 -> Compare To Constant2/1, Switch/2, Compare To Constant1/1, Compare To Constant/1
  Compare To Constant1/1 -> Delay/1
  Delay/1 -> Integrator/2
  Compare To Constant/1 -> Switch/3
  Compare To Constant2/1 -> Switch/1
  Switch/1 -> Out1/1

== system LSM_4p6U10_v01_06022022_NEW_ECC_2019a/Safety Subsystem FIELD INSTALLATION/LED STATUS/2 Blinks 3s OFF1 ==
  Enable : EnablePort  StatesWhenEnabling=reset
  Compare To Constant : simulink/Logic and Bit Operations/Compare To Constant  relop=<  const=0.25  OutDataTypeStr=boolean
  Compare To Constant1 : simulink/Logic and Bit Operations/Compare To Constant  relop=>  const=3.5  OutDataTypeStr=boolean
  Compare To Constant2 : simulink/Logic and Bit Operations/Compare To Constant  relop=<  const=0.85  OutDataTypeStr=boolean
  Constant : Constant
  Delay : Delay  DelayLength=1
  Integrator : Integrator  ExternalReset=rising  LimitOutput=on  UpperSaturationLimit=3.6  LowerSaturationLimit=0
  Switch : Switch  Criteria=u2 > Threshold  Threshold=0.5
  Out1 : Outport
  wires:
  Constant/1 -> Integrator/1
  Integrator/1 -> Compare To Constant2/1, Switch/2, Compare To Constant1/1, Compare To Constant/1
  Compare To Constant1/1 -> Delay/1
  Delay/1 -> Integrator/2
  Compare To Constant/1 -> Switch/3
  Compare To Constant2/1 -> Switch/1
  Switch/1 -> Out1/1

== system LSM_4p6U10_v01_06022022_NEW_ECC_2019a/Safety Subsystem FIELD INSTALLATION/LED STATUS/3 Blinks 3s OFF ==
  Enable : EnablePort  StatesWhenEnabling=reset
  Compare To Constant4 : simulink/Logic and Bit Operations/Compare To Constant  relop=<  const=0.25  OutDataTypeStr=boolean
  Compare To Constant5 : simulink/Logic and Bit Operations/Compare To Constant  relop=>  const=4  OutDataTypeStr=boolean
  Compare To Constant6 : simulink/Logic and Bit Operations/Compare To Constant  relop=<  const=0.85  OutDataTypeStr=boolean
  Compare To Constant7 : simulink/Logic and Bit Operations/Compare To Constant  relop=<  const=1.45  OutDataTypeStr=boolean
  Constant2 : Constant
  Delay1 : Delay  DelayLength=1
  Integrator1 : Integrator  ExternalReset=rising  LimitOutput=on  UpperSaturationLimit=4.1  LowerSaturationLimit=0
  Switch3 : Switch  Criteria=u2 > Threshold  Threshold=0.5
  Switch4 : Switch  Criteria=u2 > Threshold  Threshold=1.1
  Out1 : Outport
  wires:
  Switch3/1 -> Switch4/3
  Delay1/1 -> Integrator1/2
  Compare To Constant4/1 -> Switch3/3
  Compare To Constant5/1 -> Delay1/1
  Compare To Constant6/1 -> Switch3/1
  Integrator1/1 -> Compare To Constant7/1, Switch4/2, Compare To Constant6/1, Switch3/2, Compare To Constant5/1, Compare To Constant4/1
  Constant2/1 -> Integrator1/1
  Compare To Constant7/1 -> Switch4/1
  Switch4/1 -> Out1/1

== system LSM_4p6U10_v01_06022022_NEW_ECC_2019a/Safety Subsystem FIELD INSTALLATION/LED STATUS/3 Blinks 3s OFF1 ==
  Enable : EnablePort  StatesWhenEnabling=reset
  Compare To Constant4 : simulink/Logic and Bit Operations/Compare To Constant  relop=<  const=0.25  OutDataTypeStr=boolean
  Compare To Constant5 : simulink/Logic and Bit Operations/Compare To Constant  relop=>  const=4  OutDataTypeStr=boolean
  Compare To Constant6 : simulink/Logic and Bit Operations/Compare To Constant  relop=<  const=0.85  OutDataTypeStr=boolean
  Compare To Constant7 : simulink/Logic and Bit Operations/Compare To Constant  relop=<  const=1.45  OutDataTypeStr=boolean
  Constant2 : Constant
  Delay1 : Delay  DelayLength=1
  Integrator1 : Integrator  ExternalReset=rising  LimitOutput=on  UpperSaturationLimit=4.1  LowerSaturationLimit=0
  Switch3 : Switch  Criteria=u2 > Threshold  Threshold=0.5
  Switch4 : Switch  Criteria=u2 > Threshold  Threshold=1.1
  Out1 : Outport
  wires:
  Switch3/1 -> Switch4/3
  Delay1/1 -> Integrator1/2
  Compare To Constant4/1 -> Switch3/3
  Compare To Constant5/1 -> Delay1/1
  Compare To Constant6/1 -> Switch3/1
  Integrator1/1 -> Compare To Constant7/1, Switch4/2, Compare To Constant6/1, Switch3/2, Compare To Constant5/1, Compare To Constant4/1
  Constant2/1 -> Integrator1/1
  Compare To Constant7/1 -> Switch4/1
  Switch4/1 -> Out1/1

== system LSM_4p6U10_v01_06022022_NEW_ECC_2019a/Safety Subsystem FIELD INSTALLATION/LED STATUS/3s ON 3s OFF Slow Blink ==
  Enable : EnablePort  StatesWhenEnabling=reset
  Pulse Generator : DiscretePulseGenerator  PulseType=Time based  Period=6  PulseWidth=50
  Saturation : Saturate  UpperLimit=1  LowerLimit=0
  Out1 : Outport
  wires:
  Pulse Generator/1 -> Saturation/1
  Saturation/1 -> Out1/1

== system LSM_4p6U10_v01_06022022_NEW_ECC_2019a/Safety Subsystem FIELD INSTALLATION/LED STATUS/4 Blinks 3s OFF ==
  Enable : EnablePort  StatesWhenEnabling=reset
  Compare To Constant1 : simulink/Logic and Bit Operations/Compare To Constant  relop=<  const=2.05  OutDataTypeStr=boolean
  Compare To Constant4 : simulink/Logic and Bit Operations/Compare To Constant  relop=<  const=0.25  OutDataTypeStr=boolean
  Compare To Constant5 : simulink/Logic and Bit Operations/Compare To Constant  relop=>  const=4.5  OutDataTypeStr=boolean
  Compare To Constant6 : simulink/Logic and Bit Operations/Compare To Constant  relop=<  const=0.85  OutDataTypeStr=boolean
  Compare To Constant7 : simulink/Logic and Bit Operations/Compare To Constant  relop=<  const=1.45  OutDataTypeStr=boolean
  Constant2 : Constant
  Delay1 : Delay  DelayLength=1
  Integrator1 : Integrator  ExternalReset=rising  LimitOutput=on  UpperSaturationLimit=4.6  LowerSaturationLimit=0
  Switch1 : Switch  Criteria=u2 > Threshold  Threshold=1.8
  Switch3 : Switch  Criteria=u2 > Threshold  Threshold=0.5
  Switch4 : Switch  Criteria=u2 > Threshold  Threshold=1.1
  Out1 : Outport
  wires:
  Constant2/1 -> Integrator1/1
  Integrator1/1 -> Compare To Constant1/1, Switch1/2, Compare To Constant7/1, Switch4/2, Compare To Constant6/1, Switch3/2, Compare To Constant5/1, Compare To Constant4/1
  Compare To Constant6/1 -> Switch3/1
  Compare To Constant5/1 -> Delay1/1
  Compare To Constant4/1 -> Switch3/3
  Switch4/1 -> Switch1/3
  Switch3/1 -> Switch4/3
  Compare To Constant7/1 -> Switch4/1
  Delay1/1 -> Integrator1/2
  Switch1/1 -> Out1/1
  Compare To Constant1/1 -> Switch1/1

== system LSM_4p6U10_v01_06022022_NEW_ECC_2019a/Safety Subsystem FIELD INSTALLATION/LED STATUS/4 Blinks 3s OFF1 ==
  Enable : EnablePort  StatesWhenEnabling=reset
  Compare To Constant1 : simulink/Logic and Bit Operations/Compare To Constant  relop=<  const=2.05  OutDataTypeStr=boolean
  Compare To Constant4 : simulink/Logic and Bit Operations/Compare To Constant  relop=<  const=0.25  OutDataTypeStr=boolean
  Compare To Constant5 : simulink/Logic and Bit Operations/Compare To Constant  relop=>  const=4.5  OutDataTypeStr=boolean
  Compare To Constant6 : simulink/Logic and Bit Operations/Compare To Constant  relop=<  const=0.85  OutDataTypeStr=boolean
  Compare To Constant7 : simulink/Logic and Bit Operations/Compare To Constant  relop=<  const=1.45  OutDataTypeStr=boolean
  Constant2 : Constant
  Delay1 : Delay  DelayLength=1
  Integrator1 : Integrator  ExternalReset=rising  LimitOutput=on  UpperSaturationLimit=4.6  LowerSaturationLimit=0
  Switch1 : Switch  Criteria=u2 > Threshold  Threshold=1.8
  Switch3 : Switch  Criteria=u2 > Threshold  Threshold=0.5
  Switch4 : Switch  Criteria=u2 > Threshold  Threshold=1.1
  Out1 : Outport
  wires:
  Constant2/1 -> Integrator1/1
  Integrator1/1 -> Compare To Constant1/1, Switch1/2, Compare To Constant7/1, Switch4/2, Compare To Constant6/1, Switch3/2, Compare To Constant5/1, Compare To Constant4/1
  Compare To Constant6/1 -> Switch3/1
  Compare To Constant5/1 -> Delay1/1
  Compare To Constant4/1 -> Switch3/3
  Switch4/1 -> Switch1/3
  Switch3/1 -> Switch4/3
  Compare To Constant7/1 -> Switch4/1
  Delay1/1 -> Integrator1/2
  Switch1/1 -> Out1/1
  Compare To Constant1/1 -> Switch1/1

== system LSM_4p6U10_v01_06022022_NEW_ECC_2019a/Safety Subsystem FIELD INSTALLATION/LED STATUS/5 Blinks 3s OFF ==
  Enable : EnablePort  StatesWhenEnabling=reset
  Compare To Constant1 : simulink/Logic and Bit Operations/Compare To Constant  relop=<  const=2.05  OutDataTypeStr=boolean
  Compare To Constant2 : simulink/Logic and Bit Operations/Compare To Constant  relop=<  const=2.65  OutDataTypeStr=boolean
  Compare To Constant4 : simulink/Logic and Bit Operations/Compare To Constant  relop=<  const=0.25  OutDataTypeStr=boolean
  Compare To Constant5 : simulink/Logic and Bit Operations/Compare To Constant  relop=>  const=5.5  OutDataTypeStr=boolean
  Compare To Constant6 : simulink/Logic and Bit Operations/Compare To Constant  relop=<  const=0.85  OutDataTypeStr=boolean
  Compare To Constant7 : simulink/Logic and Bit Operations/Compare To Constant  relop=<  const=1.45  OutDataTypeStr=boolean
  Constant2 : Constant
  Delay1 : Delay  DelayLength=1
  Integrator1 : Integrator  ExternalReset=rising  LimitOutput=on  UpperSaturationLimit=5.6  LowerSaturationLimit=0
  Switch1 : Switch  Criteria=u2 > Threshold  Threshold=1.8
  Switch2 : Switch  Criteria=u2 > Threshold  Threshold=2.4
  Switch3 : Switch  Criteria=u2 > Threshold  Threshold=0.5
  Switch4 : Switch  Criteria=u2 > Threshold  Threshold=1.1
  Out1 : Outport
  wires:
  Compare To Constant1/1 -> Switch1/1
  Switch1/1 -> Switch2/3
  Delay1/1 -> Integrator1/2
  Compare To Constant7/1 -> Switch4/1
  Switch3/1 -> Switch4/3
  Switch4/1 -> Switch1/3
  Compare To Constant4/1 -> Switch3/3
  Compare To Constant5/1 -> Delay1/1
  Compare To Constant6/1 -> Switch3/1
  Integrator1/1 -> Compare To Constant4/1, Compare To Constant5/1, Switch3/2, Compare To Constant6/1, Switch4/2, Compare To Constant7/1, Switch1/2, Compare To Constant2/1, Switch2/2, Compare To Constant1/1
  Constant2/1 -> Integrator1/1
  Switch2/1 -> Out1/1
  Compare To Constant2/1 -> Switch2/1

== system LSM_4p6U10_v01_06022022_NEW_ECC_2019a/Safety Subsystem FIELD INSTALLATION/LED STATUS/ALWAYS ON ==
  Enable : EnablePort  StatesWhenEnabling=reset
  Constant1 : Constant  OutDataTypeStr=boolean
  Out1 : Outport
  wires:
  Constant1/1 -> Out1/1

== system LSM_4p6U10_v01_06022022_NEW_ECC_2019a/Thermocouples In/Read RTDs/Config Registry ==
  note: Continuous Conversion
  SPI Master Transfer2 : c280xlib/SPI Master Transfer  SPISelect=SPI_A  ClockPolarity=Rising_edge  ClockPhase=No_delay  SPIModule=uint32(0)  Mode=Master  BusSpeed=uint32(1000000)  FirstBitToTransfer=Most significant bit (MSB)  ClockMode=0  BlockFunction=Transfer  EnableRegisterAddress=on  RegisterAddress=128  OutputDataType=int8  OutputDataLength=1  DataBits=8  UseCustomSSPin=Explicit GPIO calls  ActiveLowSSPin=Active low  Pin=125
      settings: SourceProductName=Embedded Coder Support Package for Texas Instruments C2000 Processors
  Terminator1 : Terminator
  Value to Write : Constant  Value=208  OutDataTypeStr=uint16  SampleTime=-1
  wires:
  Value to Write/1 -> SPI Master Transfer2/1
  SPI Master Transfer2/1 -> Terminator1/1  "SPI_Rx_Dummy2"

== system LSM_4p6U10_v01_06022022_NEW_ECC_2019a/Thermocouples In/Read RTDs/Config Registry1 ==
  note: Continuous Conversion
  SPI Master Transfer2 : c280xlib/SPI Master Transfer  SPISelect=SPI_A  ClockPolarity=Rising_edge  ClockPhase=No_delay  SPIModule=uint32(0)  Mode=Master  BusSpeed=uint32(1000000)  FirstBitToTransfer=Most significant bit (MSB)  ClockMode=0  BlockFunction=Transfer  EnableRegisterAddress=on  RegisterAddress=128  OutputDataType=int8  OutputDataLength=1  DataBits=8  UseCustomSSPin=Explicit GPIO calls  ActiveLowSSPin=Active low  Pin=124
      settings: SourceProductName=Embedded Coder Support Package for Texas Instruments C2000 Processors
  Terminator1 : Terminator
  Value to Write : Constant  Value=208  OutDataTypeStr=uint16  SampleTime=-1
  wires:
  Value to Write/1 -> SPI Master Transfer2/1
  SPI Master Transfer2/1 -> Terminator1/1  "SPI_Rx_Dummy2"

== system LSM_4p6U10_v01_06022022_NEW_ECC_2019a/Thermocouples In/Read RTDs/Read Registry ==
  Display : Display
      settings: Format=hex (Stored Integer)
  Display1 : Display
      settings: Format=binary (Stored Integer)
  Read Configuration : Constant  Value=0  OutDataTypeStr=uint16  SampleTime=-1
  SPI Master Transfer1 : c280xlib/SPI Master Transfer  SPISelect=SPI_A  ClockPolarity=Rising_edge  ClockPhase=No_delay  SPIModule=uint32(0)  Mode=Master  BusSpeed=uint32(1000000)  FirstBitToTransfer=Most significant bit (MSB)  ClockMode=0  BlockFunction=Transfer  EnableRegisterAddress=on  RegisterAddress=0  OutputDataType=int8  OutputDataLength=1  DataBits=8  UseCustomSSPin=Explicit GPIO calls  ActiveLowSSPin=Active low  Pin=125
      settings: SourceProductName=Embedded Coder Support Package for Texas Instruments C2000 Processors
  wires:
  Read Configuration/1 -> SPI Master Transfer1/1
  SPI Master Transfer1/1 -> Display1/1, Display/1  "SPI_Rx_Dummy2"

== system LSM_4p6U10_v01_06022022_NEW_ECC_2019a/Thermocouples In/Read RTDs/Read Registry1 ==
  Display : Display
      settings: Format=hex (Stored Integer)
  Display1 : Display
      settings: Format=binary (Stored Integer)
  Read Configuration : Constant  Value=0  OutDataTypeStr=uint16  SampleTime=-1
  SPI Master Transfer1 : c280xlib/SPI Master Transfer  SPISelect=SPI_A  ClockPolarity=Rising_edge  ClockPhase=No_delay  SPIModule=uint32(0)  Mode=Master  BusSpeed=uint32(1000000)  FirstBitToTransfer=Most significant bit (MSB)  ClockMode=0  BlockFunction=Transfer  EnableRegisterAddress=on  RegisterAddress=0  OutputDataType=int8  OutputDataLength=1  DataBits=8  UseCustomSSPin=Explicit GPIO calls  ActiveLowSSPin=Active low  Pin=124
      settings: SourceProductName=Embedded Coder Support Package for Texas Instruments C2000 Processors
  wires:
  Read Configuration/1 -> SPI Master Transfer1/1
  SPI Master Transfer1/1 -> Display1/1, Display/1  "SPI_Rx_Dummy2"

== system LSM_4p6U10_v01_06022022_NEW_ECC_2019a/Thermocouples In/Read RTDs/Read Registry2 ==
  Constant : Constant  Value=0  OutDataTypeStr=uint16
  Display : Display
      settings: Format=hex (Stored Integer)
  Display1 : Display
      settings: Format=binary (Stored Integer)
  SPI Master Transfer : c280xlib/SPI Master Transfer  SPISelect=SPI_A  ClockPolarity=Rising_edge  ClockPhase=No_delay  SPIModule=uint32(0)  Mode=Master  BusSpeed=uint32(1000000)  FirstBitToTransfer=Most significant bit (MSB)  ClockMode=0  BlockFunction=Transfer  EnableRegisterAddress=on  RegisterAddress=0  OutputDataType=int8  OutputDataLength=1  DataBits=8  UseCustomSSPin=Explicit GPIO calls  ActiveLowSSPin=Active low  Pin=125
      settings: SourceProductBaseCode=TIC2000
  wires:
  SPI Master Transfer/1 -> Display1/1, Display/1  "SPI_Rx_Dummy2"
  Constant/1 -> SPI Master Transfer/1

== system LSM_4p6U10_v01_06022022_NEW_ECC_2019a/Thermocouples In/Read RTDs/Read Registry3 ==
  Constant : Constant  Value=0  OutDataTypeStr=uint16
  Display : Display
      settings: Format=hex (Stored Integer)
  Display1 : Display
      settings: Format=binary (Stored Integer)
  SPI Master Transfer : c280xlib/SPI Master Transfer  SPISelect=SPI_A  ClockPolarity=Rising_edge  ClockPhase=No_delay  SPIModule=uint32(0)  Mode=Master  BusSpeed=uint32(1000000)  FirstBitToTransfer=Most significant bit (MSB)  ClockMode=0  BlockFunction=Transfer  EnableRegisterAddress=on  RegisterAddress=0  OutputDataType=int8  OutputDataLength=1  DataBits=8  UseCustomSSPin=Explicit GPIO calls  ActiveLowSSPin=Active low  Pin=124
      settings: SourceProductBaseCode=TIC2000
  wires:
  SPI Master Transfer/1 -> Display1/1, Display/1  "SPI_Rx_Dummy2"
  Constant/1 -> SPI Master Transfer/1
